simulink model "sgMdl_IO113_20_AnalogOutputDigitalLoopback"  (R2024b)
settings: Solver=FixedStepAuto  StartTime=0.0  StopTime=inf  RelTol=1e-3  EnableMultiTasking=on
libraries: speedgoatlib_IO113 x4
Description:
  | IO113-20 - Analog Output and Digital Loopback
settings Model: ModifiedByFormat=Speedgoat  SimulationMode=external  ExtModeTrigDuration=100000  Creator=Speedgoat  LastModifiedBy=Speedgoat
settings SolverCC: ConcurrentTasks=on  AlgebraicLoopSolver=TrustRegion  PositivePriorityOrder=on  InsertRTBMode=Never (minimum delay)
settings DataIOCC: SaveFormat=Array  SaveState=on  SignalLoggingName=logsOut
settings OptimizationCC: BlockReduction=off  BooleanDataType=off  OptimizeBlockIOStorage=off  BufferReuse=off  ReuseModelBlockBuffer=off  GlobalBufferReuse=off  ExpressionFolding=off  LocalBlockOutputs=off  InitFltsAndDblsToZero=on  OptimizeDataStoreBuffers=off  BusAssignmentInplaceUpdate=off
settings DebuggingCC: SaveWithParameterizedLinksMsg=none  UnderspecifiedInitializationDetection=Classic  MergeDetectMultiDrivingBlocksExec=none  CheckExecutionContextPreStartOutputMsg=on  SignalResolutionControl=TryResolveAllWithWarning  TasksWithSamePriorityMsg=none  UnconnectedInputMsg=warning  UnconnectedOutputMsg=warning  UnconnectedLineMsg=warning  SFUnexpectedBacktrackingDiag=warning  SFNoUnconditionalDefaultTransitionDiag=warning  SFExecutionAtInitializationDiag=none  ArithmeticOperatorsInVariantConditions=warning
settings HardwareCC: ProdBitPerLong=64  ProdLongLongMode=on  ProdHWDeviceType=Intel->x86-64 (Linux 64)
settings ModelReferenceCC: EnableRefExpFcnMdlSchedulingChecks=on  PropagateSignalLabelsOutOfModel=off
settings SFSimCC: SimUseLocalCustomCode=off  SimTargetLang=C++
settings RTWCC: Description=Speedgoat Real-Time Target Machine  SystemTargetFile=speedgoat.tlc  TemplateMakefile=slrealtime_default_tmf  RTWUseLocalCustomCode=off  Toolchain=Simulink Real-Time Toolchain  BuildConfiguration=Faster Runs  TargetLang=C++  GPUComputeCapability=3.5  DLArmComputeVersion=19.05
settings CodeAppCC: StateflowObjectComments=on
settings SimulinkRealTimeTargetCC: SubcomponentCodeInterfacePackaging=Reusable function  MATLABClassNameForMDSCustomization=Simulink.SoftwareTarget.GRTCustomization  InstructionSetFMA=off  LogToMDFFile=off  SLRTFileLogMaxRuns=10  UseGCCFastMath=on
settings ConfigComp: CovMetricSettings=dw  CovSaveCumulativeToWorkspaceVar=on  CovSaveSingleToWorkspaceVar=on  CovExternalEMLEnable=off  CovSFcnEnable=off  CovBoundaryAbsTol=1.0e-5

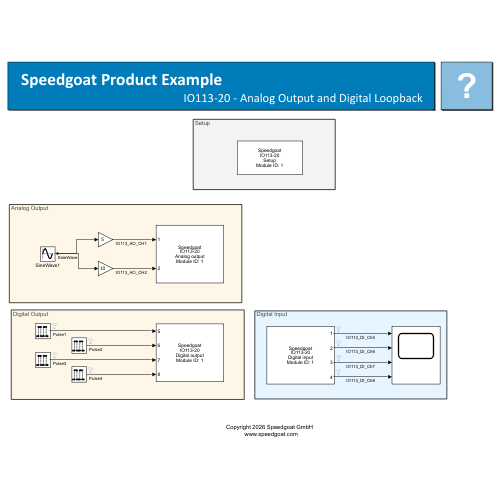
[thumbnail: Simulink's stored preview of the top-level diagram]
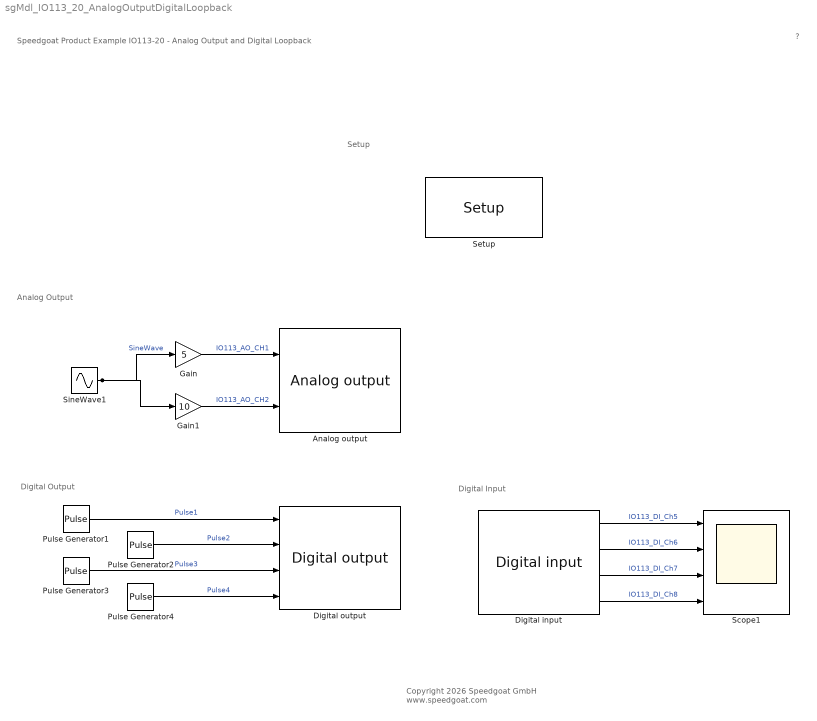
== system sgMdl_IO113_20_AnalogOutputDigitalLoopback ==
  note: Digital Input
  note: Digital Output
  note: Analog Output
  note: Setup
  note: Speedgoat Product Example
      | IO113-20 - Analog Output and Digital Loopback
  note: ?
  note: Copyright 2026 Speedgoat GmbH
      |  www.speedgoat.com
  "Analog output " : speedgoatlib_IO113/IO113-20/Analog output   parModuleId=1  parSampleTime=-1  parPciSlot=-1  parDacChannels=[1 2]  parModuleType=1  parDacRangeA=1  parDacRangeB=1  parDacInitValues=[0 0]  parDacResets=[1 1]
      settings: SourceProductName=Simulink Real-Time: Speedgoat I/O Blockset
  "Digital input " : speedgoatlib_IO113/IO113-20/Digital input   parModuleId=1  parSampleTime=-1  parPciSlot=-1  parDiChannels=[5 6 7 8]
      settings: SourceProductName=Simulink Real-Time: Speedgoat I/O Blockset
  "Digital output " : speedgoatlib_IO113/IO113-20/Digital output   parModuleId=1  parSampleTime=-1  parPciSlot=-1  parDoChannels=[1 2 3 4]  parDoInitValues=[0 0 0 0]  parDoResets=[1 1 1 1]
      settings: SourceProductName=Simulink Real-Time: Speedgoat I/O Blockset
  Gain : Gain  Gain=5
  Gain1 : Gain  Gain=10
  Pulse Generator1 : DiscretePulseGenerator  Period=10  PulseWidth=5  SampleTime=-1
  Pulse Generator2 : DiscretePulseGenerator  Period=20  PulseWidth=5  SampleTime=-1
  Pulse Generator3 : DiscretePulseGenerator  Period=20  PulseWidth=10  SampleTime=-1
  Pulse Generator4 : DiscretePulseGenerator  Period=40  PulseWidth=10  SampleTime=-1
  Scope1 : Scope  NumInputPorts=4
  "Setup " : speedgoatlib_IO113/IO113-20/Setup   parPciSlot=-1  parModuleId=1  parTriggerSignal=TTL  parModuleType=+-10 V and +-5 V  parCalibration=on  parFilter=off  parDacChannels=[1 2]  parDacChannel1=on  parDacChannel2=on  parDacChannel3=off  parDacChannel4=off  parDacChannel5=off  parDacChannel6=off  parDacChannel7=off  parDacChannel8=off  parDaMode=Single-ended  parDacInitValues=[0 0]  parDacRangeA=+-10 V  parDacResets=[1 1]  parDacRangeB=+-5 V  parDacInitValue1=0  parDacReset1=on  parDacInitValue2=0  parDacReset2=on  parDacInitValue3=0  parDacReset3=on  parDacInitValue4=0  parDacReset4=on  parDacInitValue5=0  parDacReset5=on  parDacInitValue6=0  parDacReset6=on  parDacInitValue7=0  parDacReset7=on  parDacInitValue8=0  parDacReset8=on  parDiChannels=[3 4]  parDoChannels=[1 2 3 4]  parDioFirstControl=1  parDioSecondControl=0  parDioChannel1=Output  parDioChannel2=Input  parDoInitValues=[0 0 0 0]  parDoResets=[1 1 1 1]  parDoInitValue1=0  parDoReset1=on  parDoInitValue2=0  parDoReset2=on  parDoInitValue3=0  parDoReset3=on  parDoInitValue4=0  parDoReset4=on  parDoInitValue5=0  parDoReset5=on  parDoInitValue6=0  parDoReset6=on  parDoInitValue7=0  parDoReset7=on  parDoInitValue8=0  parDoReset8=on
      settings: SourceProductName=Simulink Real-Time: Speedgoat I/O Blockset
  SineWave1 : Sin  Frequency=2*pi  Samples=50
  wires:
  Gain/1 -> "Analog output "/1  "IO113_AO_CH1"
  Gain1/1 -> "Analog output "/2  "IO113_AO_CH2"
  SineWave1/1 -> Gain/1, Gain1/1  "SineWave"
  Pulse Generator1/1 -> "Digital output "/1  "Pulse1"
  "Digital input "/4 -> Scope1/4  "IO113_DI_Ch8"
  "Digital input "/3 -> Scope1/3  "IO113_DI_Ch7"
  "Digital input "/2 -> Scope1/2  "IO113_DI_Ch6"
  "Digital input "/1 -> Scope1/1  "IO113_DI_Ch5"
  Pulse Generator2/1 -> "Digital output "/2  "Pulse2"
  Pulse Generator3/1 -> "Digital output "/3  "Pulse3"
  Pulse Generator4/1 -> "Digital output "/4  "Pulse4"
